simulink model "sensor"  (R2022b)
settings: Solver=FixedStepDiscrete  StartTime=0.0  StopTime=10.0  RelTol=1e-3
settings Model: Creator=lcx19  LastModifiedBy=lcx19

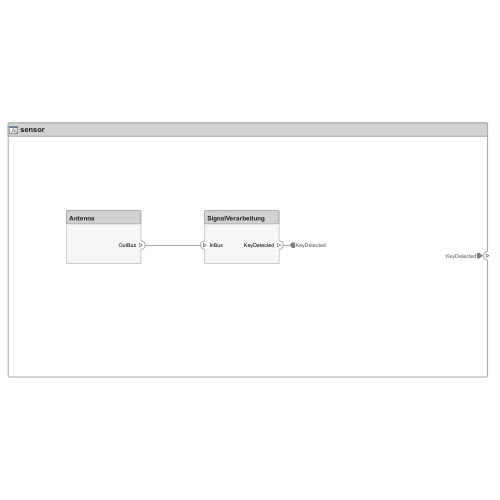
[thumbnail: Simulink's stored preview of the top-level diagram]
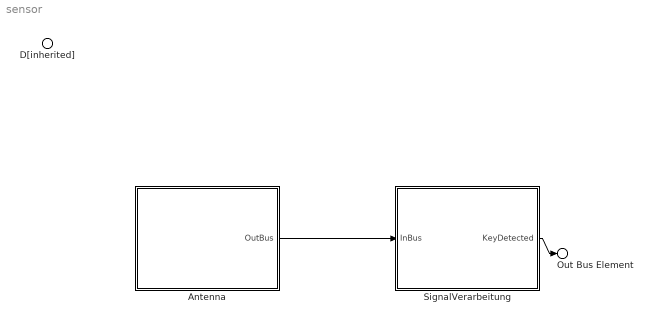
== system sensor ==
  D[inherited] : Inport  OutputFunctionCall=on
  Antenna : Subsystem
      settings: PortSchema="{\"entries\":[{\"content\":{\"headerSize\":26,\"margin\":15,\"minimumSpacing\":25,\"sides\":[{\"content\":{\"connectorIds\":[]},\"type\":\"ConnectorPlacement.EquallySpacedRectSide\",\"uuid\":\"b7c7e327-1f1f-4c3c-8395-c1654c938907\"},{\"content\":{\"connectorIds\":[\"Out1\"],\"side\":\"RIGHT\"},\"type\":\"ConnectorPlacement.EquallySpacedRectSide\",\"uuid\":\"66bc2f54-eb79-4f92-ad10-538e1a27c73a\"},{\"content\":{\"connectorIds\":[],\"side\":\"TOP\"},\"type\":\"ConnectorPlacement.EquallySpacedRectSide\",\"uuid\":\"6c491a77-0a9f-4c26-92d1-b5454ed3d912\"}]},\"type\":\"ConnectorPlacement.EquallySpacedConnector\",\"uuid\":\"9ab7e123-0a39-41c9-a0e0-1e5de1cb6ec8\"}],\"packageUris\":[\"http://schema.mathworks.com/mf0/Connector/R2020b\"],\"version\":\"1.0\"}"
  SignalVerarbeitung : Subsystem
      settings: PortSchema="{\"entries\":[{\"content\":{\"headerSize\":26,\"margin\":15,\"minimumSpacing\":25,\"sides\":[{\"content\":{\"connectorIds\":[\"In1\"]},\"type\":\"ConnectorPlacement.EquallySpacedRectSide\",\"uuid\":\"b7c7e327-1f1f-4c3c-8395-c1654c938907\"},{\"content\":{\"connectorIds\":[\"Out1\"],\"side\":\"RIGHT\"},\"type\":\"ConnectorPlacement.EquallySpacedRectSide\",\"uuid\":\"66bc2f54-eb79-4f92-ad10-538e1a27c73a\"},{\"content\":{\"connectorIds\":[],\"side\":\"TOP\"},\"type\":\"ConnectorPlacement.EquallySpacedRectSide\",\"uuid\":\"6c491a77-0a9f-4c26-92d1-b5454ed3d912\"}]},\"type\":\"ConnectorPlacement.EquallySpacedConnector\",\"uuid\":\"9ab7e123-0a39-41c9-a0e0-1e5de1cb6ec8\"}],\"packageUris\":[\"http://schema.mathworks.com/mf0/Connector/R2020b\"],\"version\":\"1.0\"}"
  Out Bus Element : Outport  PortName=KeyDetected
  wires:
  Antenna/1(OutBus) -> SignalVerarbeitung/1(InBus)
  SignalVerarbeitung/1(KeyDetected) -> Out Bus Element/1

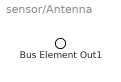
== system sensor/Antenna ==
  Bus Element Out1 : Outport  PortName=OutBus

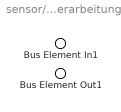
== system sensor/SignalVerarbeitung ==
  Bus Element In1 : Inport  PortName=InBus
  Bus Element Out1 : Outport  PortName=KeyDetected
